simulink model "plant"  (R2022b)
settings: Solver=FixedStepAuto  StartTime=0.0  StopTime=10  FixedStep=0.00001  RelTol=1e-3
values from neighbouring files (symbols this model uses):
  ai = 0:0.03:20    [gain_schedule_co.m]
  Mi = 1.5:0.01:3    [gain_schedule_co.m]
undefined symbols (not defined in the file or in its folder): a_G0, a_G1, a_G2, a_G3, a_H0, a_H1, a_H2, a_H3, b_G0, b_G1, b_G2, b_G3, b_G4, b_H0, b_H1, b_H2, b_H3, b_H4, sigbuilder_block
libraries: cstblocks x2, SignalEditorBlockLib x1
settings Model: Creator=tomkeen  LastModifiedBy=tomkeen
settings SolverCC: AlgebraicLoopSolver=TrustRegion
settings DebuggingCC: UnconnectedInputMsg=warning  UnconnectedOutputMsg=warning  UnconnectedLineMsg=warning  SFMachineParentedDataDiag=warning
settings ModelReferenceCC: EnableRefExpFcnMdlSchedulingChecks=on
settings RTWCC: DLArmComputeVersion=19.05

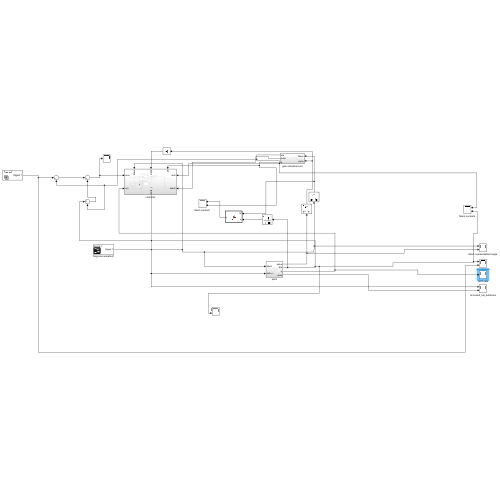
[thumbnail: Simulink's stored preview of the top-level diagram]
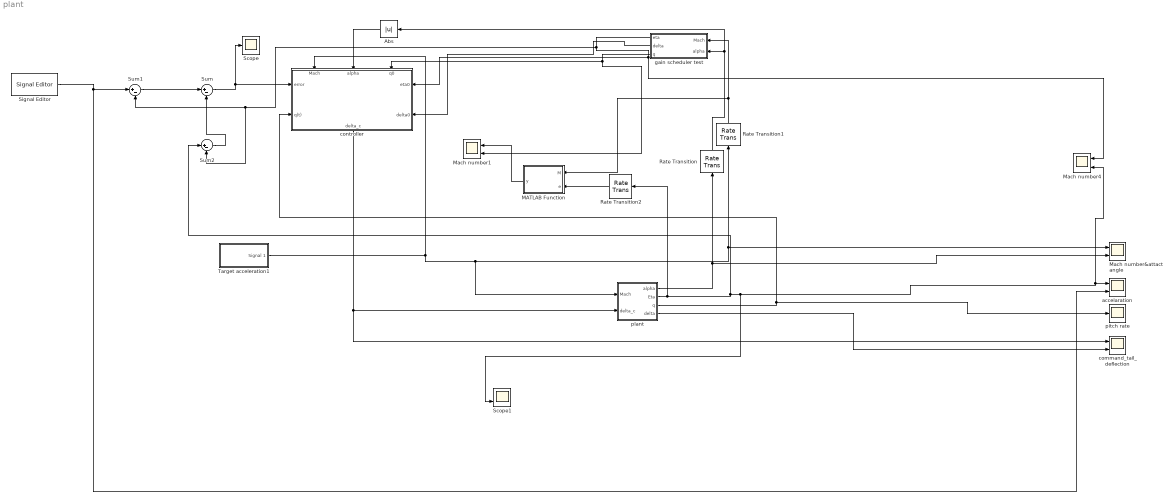
== system plant ==
  " pitch rate" : Scope
  Abs : Abs  SaturateOnIntegerOverflow=off
  MATLAB Function : MATLAB Function  TreatAsAtomicUnit=on
  Mach number&attact angle : Scope  NumInputPorts=2
  Mach number1 : Scope  NumInputPorts=2
  Mach number4 : Scope  NumInputPorts=2
  Rate Transition : RateTransition  OutPortSampleTime=0.001
  Rate Transition1 : RateTransition  OutPortSampleTime=0.001
  Rate Transition2 : RateTransition  OutPortSampleTime=0.0001
  Scope : Scope
  Scope1 : Scope  NumInputPorts=2
  Signal Editor : SignalEditorBlockLib/Signal Editor  FileName=signal.mat  ActiveScenario=Scenario  ActiveSignal=Signal 1  IsBus=off  OutputBusObjectStr=Bus: BusObject  SampleTime=0  Interpolate=off  ZeroCross=off  OutputAfterFinalValue=Setting to zero  Unit=inherit  PreserveSignalName=on
  Sum : Sum  Inputs=|+-
  Sum1 : Sum  Inputs=|+-
  Sum2 : Sum  Inputs=|+-
  Target acceleration1 : Subsystem  Tag=STV Subsys  LoadFcn=sigbuilder_block('load',[278.5 464.5 513.5 322.5 ]);  StartFcn=sigbuilder_block('start');  StopFcn=sigbuilder_block('stop');  ClipboardFcn=sigbuilder_block('clipboard');  mask(Sigbuilder block){tuvar=[0:10]}
      mask help: Simulink:masks:SigbuilderBlock_MD
      mask init:
      | if ~strcmp(get_param(bdroot(gcbh),'SimulationStatus'),'stopped') tuvar = sigbuilder_block('maskInit'); end
      settings: CopyFcn=sigbuilder_block('copy');  DeleteFcn=sigbuilder_block('delete');  ModelCloseFcn=sigbuilder_block('modelClose');  PreSaveFcn=sigbuilder_block('preSave');  PauseFcn=sigbuilder_block('pause');  ContinueFcn=sigbuilder_block('continue');  NameChangeFcn=sigbuilder_block('namechange');  OpenFcn=sigbuilder_block('open',[221 107.5 550.5 322.5 ]);  CloseFcn=sigbuilder_block('close');
      mask Display: plot(0, 0, 100, 100,[2, 2, 32, 32, 2], [68, 8, 8, 68, 68],[32, 2], [38, 38], [32, 19, 2],[53, 60, 44], [32, 17, 17, 2],[16, 16, 31, 31]);txt = getActiveGroup(gcbh);text(2, 100, txt,'verticalAlignment', 'top');
  accelaration : Scope  NumInputPorts=2
  command_tail_deflection : Scope  NumInputPorts=2
  controller : Subsystem
      settings: PortSchema="{\"entries\":[{\"content\":{\"sides\":[{\"content\":{\"connectorIds\":[\"In1\",\"In2\"]},\"type\":\"ConnectorPlacement.EquallySpacedRectSide\",\"uuid\":\"ccbd3968-3c34-4172-8982-2717baa6aaec\"},{\"content\":{\"connectorIds\":[\"In6\",\"In7\"],\"side\":\"RIGHT\"},\"type\":\"ConnectorPlacement.EquallySpacedRectSide\",\"uuid\":\"ff48a950-eb2b-4faf-a742-71355e33462e\"},{\"content\":{\"connectorIds\":[\"In3\",\"In4\",\"In5\"],\"side\":\"TOP\"},\"type\":\"ConnectorPlacement.EquallySpacedRectSide\",\"uuid\":\"543e7319-a8cd-4270-affa-865af0d15bcc\"},{\"content\":{\"connectorIds\":[\"Out1\"],\"side\":\"BOTTOM\"},\"type\":\"ConnectorPlacement.EquallySpacedRectSide\",\"uuid\":\"59242803-d082-430c-87a9-b5e2615a3fae\"}]},\"type\":\"ConnectorPlacement.EquallySpacedConnector\",\"uuid\":\"c7654354-e930-4276-ba78-f9f6fb08bf2c\"}],\"packageUris\":[\"http://schema.mathworks.com/mf0/Connector/R2020b\"],\"version\":\"1.0\"}"
  gain scheduler test : Subsystem
  plant : Subsystem
  wires:
  Target acceleration1/1(Signal 1) -> Rate Transition1/1, Mach number&attact angle/1, plant/1(Mach), controller/5(Mach)
  plant/2(Eta) -> Rate Transition2/1, Sum2/1, Scope1/2, Mach number4/2, accelaration/1
  plant/3(q) -> controller/7(q(t)), " pitch rate"/1
  plant/4(delta) -> command_tail_deflection/2
  gain scheduler test/2(delta) -> controller/2(delta0)
  gain scheduler test/3(q) -> controller/3(q0), Mach number1/2
  gain scheduler test/1(eta) -> controller/1(eta0), Mach number4/1, Sum2/2, Sum1/2
  Sum/1 -> Scope/1, controller/6(error)
  controller/1(delta_c) -> command_tail_deflection/1, plant/2(delta_c)
  Signal Editor/1 -> accelaration/2, Sum1/1
  Sum1/1 -> Sum/1
  Sum2/1 -> Sum/2
  Rate Transition/1 -> gain scheduler test/2(alpha), Abs/1
  Rate Transition1/1 -> gain scheduler test/1(Mach), MATLAB Function/1(M)
  plant/1(alpha) -> Rate Transition/1, Mach number&attact angle/2
  MATLAB Function/1(y) -> Mach number1/1
  Rate Transition2/1 -> MATLAB Function/2(e)
  Abs/1 -> controller/4(alpha)

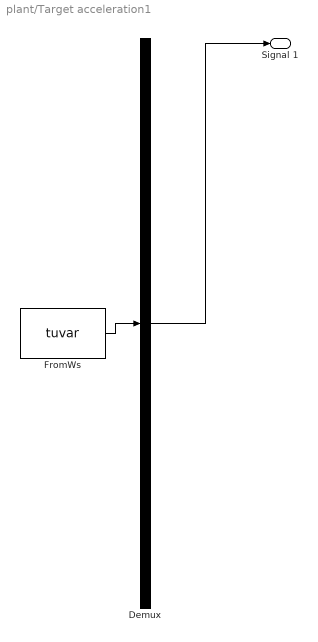
== system plant/Target acceleration1 ==
  Demux : Demux  Tag=STV Demux  Outputs=1
      settings: DisplayOption=none
  FromWs : FromWorkspace  Tag=STV FromWs  VariableName=tuvar
      SigBuilderData=|
      | common.afterFinalStr = 'Extrapolate'
      | common.sampleTime = 0
      | dataSet.timeRange = [0 10]
      | dataSet.name = 'Group 1'
      | sbobj.Groups.Name = 'Group 1'
      | sbobj.Groups.Signals.Name = 'Signal 1'
      | sbobj.Groups.Signals.XData = [0 10]
      | sbobj.Groups.Signals.YData = [2.69 2.48816513761]
  Signal 1 : Outport  Tag=STV Outport
  wires:
  Demux/1 -> Signal 1/1
  FromWs/1 -> Demux/1

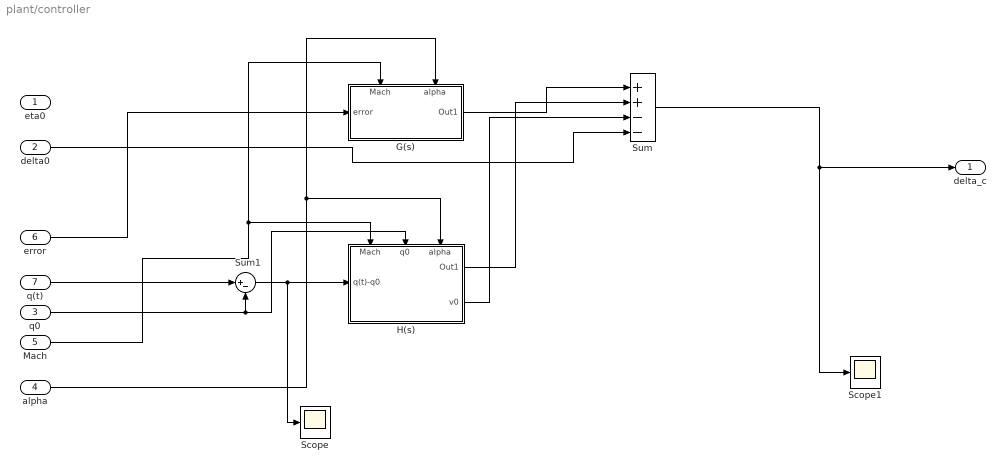
== system plant/controller ==
  eta0 : Inport
  delta0 : Inport  Port=2
  q0 : Inport  Port=3
  alpha : Inport  Port=4
  Mach : Inport  Port=5
  error : Inport  Port=6
  q(t) : Inport  Port=7
  G(s) : Subsystem
      settings: PortSchema="{\"entries\":[{\"content\":{\"sides\":[{\"content\":{\"connectorIds\":[\"In1\"]},\"type\":\"ConnectorPlacement.EquallySpacedRectSide\",\"uuid\":\"89c4dd89-01f0-41d8-90e7-82360ec46edc\"},{\"content\":{\"connectorIds\":[\"Out1\"],\"side\":\"RIGHT\"},\"type\":\"ConnectorPlacement.EquallySpacedRectSide\",\"uuid\":\"293521c5-f39c-474b-9224-6fe6832128f5\"},{\"content\":{\"connectorIds\":[\"In2\",\"In3\"],\"side\":\"TOP\"},\"type\":\"ConnectorPlacement.EquallySpacedRectSide\",\"uuid\":\"cd72ac66-ac52-4d27-85e4-85a309f5cd1a\"}]},\"type\":\"ConnectorPlacement.EquallySpacedConnector\",\"uuid\":\"92567c15-3faa-47ed-b120-3a292a4ff95e\"}],\"packageUris\":[\"http://schema.mathworks.com/mf0/Connector/R2020b\"],\"version\":\"1.0\"}"
  H(s) : Subsystem
      settings: PortSchema="{\"entries\":[{\"content\":{\"sides\":[{\"content\":{\"connectorIds\":[\"In1\"]},\"type\":\"ConnectorPlacement.EquallySpacedRectSide\",\"uuid\":\"89c4dd89-01f0-41d8-90e7-82360ec46edc\"},{\"content\":{\"connectorIds\":[\"Out1\",\"Out2\"],\"side\":\"RIGHT\"},\"type\":\"ConnectorPlacement.EquallySpacedRectSide\",\"uuid\":\"293521c5-f39c-474b-9224-6fe6832128f5\"},{\"content\":{\"connectorIds\":[\"In2\",\"In3\",\"In4\"],\"side\":\"TOP\"},\"type\":\"ConnectorPlacement.EquallySpacedRectSide\",\"uuid\":\"cd72ac66-ac52-4d27-85e4-85a309f5cd1a\"}]},\"type\":\"ConnectorPlacement.EquallySpacedConnector\",\"uuid\":\"92567c15-3faa-47ed-b120-3a292a4ff95e\"}],\"packageUris\":[\"http://schema.mathworks.com/mf0/Connector/R2020b\"],\"version\":\"1.0\"}"
  Scope : Scope
  Scope1 : Scope
  Sum : Sum  Inputs=|++--
  Sum1 : Sum  Inputs=|+-
  delta_c : Outport
  wires:
  G(s)/1(Out1) -> Sum/1
  H(s)/1(Out1) -> Sum/2
  Sum/1 -> Scope1/1, delta_c/1
  alpha/1 -> G(s)/3(alpha), H(s)/4(alpha)
  Mach/1 -> G(s)/2(Mach), H(s)/2(Mach)
  error/1 -> G(s)/1(error)
  q(t)/1 -> Sum1/1
  Sum1/1 -> Scope/1, H(s)/1(q(t)-q0)
  q0/1 -> H(s)/3(q0), Sum1/2
  H(s)/2(v0) -> Sum/3
  delta0/1 -> Sum/4

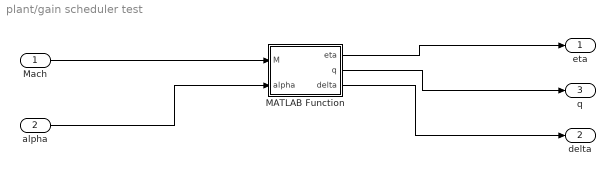
== system plant/gain scheduler test ==
  Mach : Inport
  alpha : Inport  Port=2
  MATLAB Function : MATLAB Function  TreatAsAtomicUnit=on
  eta : Outport
  delta : Outport  Port=2
  q : Outport  Port=3
  wires:
  Mach/1 -> MATLAB Function/1(M)
  alpha/1 -> MATLAB Function/2(alpha)
  MATLAB Function/1(eta) -> eta/1
  MATLAB Function/2(q) -> q/1
  MATLAB Function/3(delta) -> delta/1

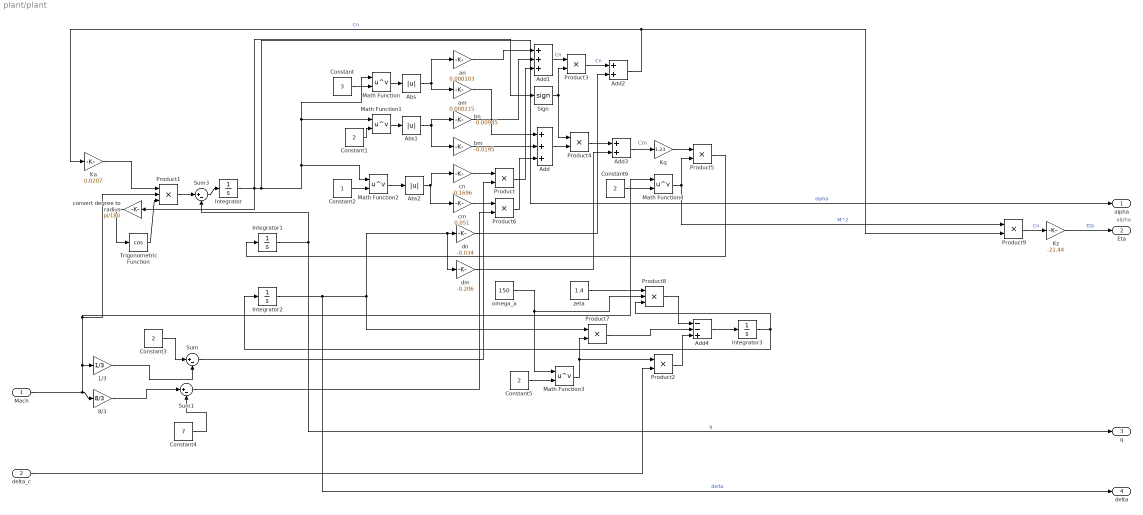
== system plant/plant ==
  note: alpha
  note: Cm
  Mach : Inport
  delta_c : Inport  Port=2
  1/3 : Gain  Gain=1/3
  8/3 : Gain  Gain=8/3
  Abs : Abs  SaturateOnIntegerOverflow=off
  Abs1 : Abs  SaturateOnIntegerOverflow=off
  Abs2 : Abs  SaturateOnIntegerOverflow=off
  Add : Sum  Inputs=+++
  Add1 : Sum  Inputs=+++
  Add2 : Sum
  Add3 : Sum
  Add4 : Sum  Inputs=--+
  Constant : Constant  Value=3
  Constant{1,3,5..6} (4 alike) : Constant  Value=2
  Constant2 : Constant
  Constant4 : Constant  Value=7
  Integrator{,1..3} (4 alike) : Integrator
  Ka : Gain  Gain=0.0207
  Kq : Gain  Gain=1.23
  Kz : Gain  Gain=-21.44
  Math Function{,1..4} (5 alike) : Math  Operator=pow
  Product{,2..7,9} (8 alike) : Product
  Product1 : Product  Inputs=3
  Product8 : Product  Inputs=3
  Sign : Signum
  Sum : Sum  Inputs=|+-
  Sum1 : Sum  Inputs=|+-
  Sum3 : Sum  Inputs=|+-
  Trigonometric Function : Trigonometry  Operator=cos
  am : Gain  Gain=0.000215
  an : Gain  Gain=0.000103
  bm : Gain  Gain=-0.0195
  bn : Gain  Gain=-0.00945
  cm : Gain  Gain=0.051
  cn : Gain  Gain=-0.1696
  convert degree to radius : Gain  Gain=pi/180
  dm : Gain  Gain=-0.206
  dn : Gain  Gain=-0.034
  omega_a : Constant  Value=150
  zeta : Constant  Value=1.4
  alpha : Outport
  Eta : Outport  Port=2
  q : Outport  Port=3
  delta : Outport  Port=4
  wires:
  Sign/1 -> Product4/1, Product3/2
  Product/1 -> Add1/3
  Integrator3/1 -> Integrator2/1, Product8/3
  Integrator1/1 -> q/1, Sum3/2  "q"
  Mach/1 -> Math Function4/1, Product1/2, 1/3/1, 8/3/1
  Sum/1 -> Product/2
  dm/1 -> Add3/2
  Add2/1 -> Product9/2, Ka/1  "Cn"
  Integrator2/1 -> delta/1, Product7/1, dm/1, dn/1  "delta"
  am/1 -> Add/1
  Abs/1 -> an/1, am/1
  Integrator/1 -> Sign/1, alpha/1, Math Function/1, Math Function1/1, Math Function2/1, convert degree to radius/1  "alpha"
  Abs1/1 -> bm/1, bn/1
  Ka/1 -> Product1/1
  Product4/1 -> Add3/1
  Add3/1 -> Kq/1
  Constant5/1 -> Math Function3/2
  Product5/1 -> Integrator1/1
  1/3/1 -> Sum/2
  Abs2/1 -> cm/1, cn/1
  cm/1 -> Product6/1
  Constant/1 -> Math Function/2
  zeta/1 -> Product8/1
  Constant3/1 -> Sum/1
  Product7/1 -> Add4/2
  Constant6/1 -> Math Function4/2
  an/1 -> Add1/1
  Product6/1 -> Add/3
  Constant4/1 -> Sum1/2
  bm/1 -> Add/2
  dn/1 -> Add2/2
  Math Function2/1 -> Abs2/1
  Add1/1 -> Product3/1  "Cn"
  Product1/1 -> Sum3/1
  Math Function1/1 -> Abs1/1
  Sum3/1 -> Integrator/1
  Math Function3/1 -> Product2/1, Product7/2
  omega_a/1 -> Product8/2, Math Function3/1
  Math Function/1 -> Abs/1
  Constant2/1 -> Math Function2/2
  cn/1 -> Product/1
  Add/1 -> Product4/2
  Trigonometric Function/1 -> Product1/3
  Product3/1 -> Add2/1  "Cn"
  bn/1 -> Add1/2
  delta_c/1 -> Product2/2
  8/3/1 -> Sum1/1
  Sum1/1 -> Product6/2
  Product8/1 -> Add4/1
  Product2/1 -> Add4/3
  Constant1/1 -> Math Function1/2
  Product9/1 -> Kz/1  "Cn"
  Math Function4/1 -> Product9/1, Product5/2  "M^2"
  Add4/1 -> Integrator3/1
  Kq/1 -> Product5/1
  Kz/1 -> Eta/1  "Eta"
  convert degree to radius/1 -> Trigonometric Function/1

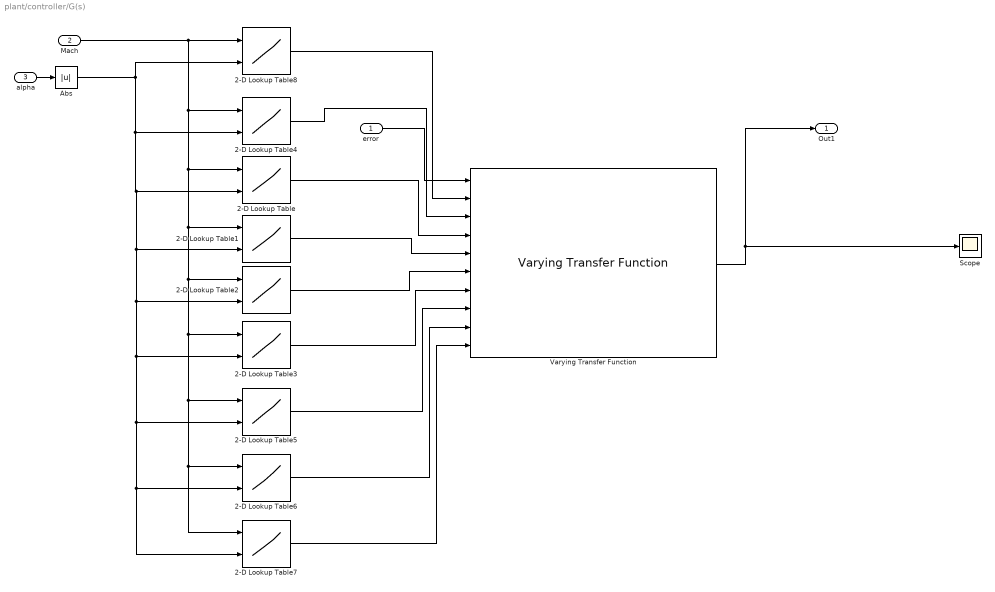
== system plant/controller/G(s) ==
  error : Inport
  Mach : Inport  Port=2
  alpha : Inport  Port=3
  2-D Lookup Table : Lookup_n-D  LookupTableObject=''  BreakpointsForDimension1=Mi  BreakpointsForDimension2=ai  BreakpointsForDimension1FirstPoint=10  BreakpointsForDimension2FirstPoint=10  BreakpointsForDimension1Spacing=12  BreakpointsForDimension2Spacing=12  IndexSearchMethod=Evenly spaced points  Table=b_G1  InterpMethod=Flat  DiagnosticForOutOfRangeInput=Error  InternalRulePriority=Speed  RndMeth=Simplest
      settings: InputPortMap=u0,u1
  2-D Lookup Table1 : Lookup_n-D  LookupTableObject=''  BreakpointsForDimension1=Mi  BreakpointsForDimension2=ai  BreakpointsForDimension1FirstPoint=10  BreakpointsForDimension2FirstPoint=10  BreakpointsForDimension1Spacing=12  BreakpointsForDimension2Spacing=12  IndexSearchMethod=Evenly spaced points  Table=a_G1  InterpMethod=Flat  DiagnosticForOutOfRangeInput=Error  InternalRulePriority=Speed  RndMeth=Simplest
      settings: InputPortMap=u0,u1
  2-D Lookup Table2 : Lookup_n-D  LookupTableObject=''  BreakpointsForDimension1=Mi  BreakpointsForDimension2=ai  BreakpointsForDimension1FirstPoint=10  BreakpointsForDimension2FirstPoint=10  BreakpointsForDimension1Spacing=12  BreakpointsForDimension2Spacing=12  IndexSearchMethod=Evenly spaced points  Table=b_G2  InterpMethod=Flat  DiagnosticForOutOfRangeInput=Error  InternalRulePriority=Speed  RndMeth=Simplest
      settings: InputPortMap=u0,u1
  2-D Lookup Table3 : Lookup_n-D  LookupTableObject=''  BreakpointsForDimension1=Mi  BreakpointsForDimension2=ai  BreakpointsForDimension1FirstPoint=10  BreakpointsForDimension2FirstPoint=10  BreakpointsForDimension1Spacing=12  BreakpointsForDimension2Spacing=12  IndexSearchMethod=Evenly spaced points  Table=a_G2  InterpMethod=Flat  DiagnosticForOutOfRangeInput=Error  InternalRulePriority=Speed  RndMeth=Simplest
      settings: InputPortMap=u0,u1
  2-D Lookup Table4 : Lookup_n-D  LookupTableObject=''  BreakpointsForDimension1=Mi  BreakpointsForDimension2=ai  BreakpointsForDimension1FirstPoint=10  BreakpointsForDimension2FirstPoint=10  BreakpointsForDimension1Spacing=12  BreakpointsForDimension2Spacing=12  IndexSearchMethod=Evenly spaced points  Table=a_G0  InterpMethod=Flat  DiagnosticForOutOfRangeInput=Error  InternalRulePriority=Speed  RndMeth=Simplest
      settings: InputPortMap=u0,u1
  2-D Lookup Table5 : Lookup_n-D  LookupTableObject=''  BreakpointsForDimension1=Mi  BreakpointsForDimension2=ai  BreakpointsForDimension1FirstPoint=10  BreakpointsForDimension2FirstPoint=10  BreakpointsForDimension1Spacing=12  BreakpointsForDimension2Spacing=12  IndexSearchMethod=Evenly spaced points  Table=b_G3  InterpMethod=Flat  DiagnosticForOutOfRangeInput=Error  InternalRulePriority=Speed  RndMeth=Simplest
      settings: InputPortMap=u0,u1
  2-D Lookup Table6 : Lookup_n-D  LookupTableObject=''  BreakpointsForDimension1=Mi  BreakpointsForDimension2=ai  BreakpointsForDimension1FirstPoint=10  BreakpointsForDimension2FirstPoint=10  BreakpointsForDimension1Spacing=12  BreakpointsForDimension2Spacing=12  IndexSearchMethod=Evenly spaced points  Table=a_G3  InterpMethod=Flat  DiagnosticForOutOfRangeInput=Error  InternalRulePriority=Speed  RndMeth=Simplest
      settings: InputPortMap=u0,u1
  2-D Lookup Table7 : Lookup_n-D  LookupTableObject=''  BreakpointsForDimension1=Mi  BreakpointsForDimension2=ai  BreakpointsForDimension1FirstPoint=10  BreakpointsForDimension2FirstPoint=10  BreakpointsForDimension1Spacing=12  BreakpointsForDimension2Spacing=12  IndexSearchMethod=Evenly spaced points  Table=b_G4  InterpMethod=Flat  DiagnosticForOutOfRangeInput=Error  InternalRulePriority=Speed  RndMeth=Simplest
      settings: InputPortMap=u0,u1
  2-D Lookup Table8 : Lookup_n-D  LookupTableObject=''  BreakpointsForDimension1=Mi  BreakpointsForDimension2=ai  BreakpointsForDimension1FirstPoint=10  BreakpointsForDimension2FirstPoint=10  BreakpointsForDimension1Spacing=12  BreakpointsForDimension2Spacing=12  IndexSearchMethod=Evenly spaced points  Table=b_G0  InterpMethod=Flat  DiagnosticForOutOfRangeInput=Error  InternalRulePriority=Speed  RndMeth=Simplest
      settings: InputPortMap=u0,u1
  Abs : Abs  SaturateOnIntegerOverflow=off
  Scope : Scope
  Varying Transfer Function : cstblocks/Linear Parameter Varying/Varying Transfer Function  N=4
  Out1 : Outport
  wires:
  error/1 -> Varying Transfer Function/1
  Varying Transfer Function/1 -> Out1/1, Scope/1
  2-D Lookup Table6/1 -> Varying Transfer Function/9
  2-D Lookup Table7/1 -> Varying Transfer Function/10
  2-D Lookup Table5/1 -> Varying Transfer Function/8
  2-D Lookup Table3/1 -> Varying Transfer Function/7
  2-D Lookup Table2/1 -> Varying Transfer Function/6
  2-D Lookup Table1/1 -> Varying Transfer Function/5
  2-D Lookup Table/1 -> Varying Transfer Function/4
  2-D Lookup Table4/1 -> Varying Transfer Function/3
  2-D Lookup Table8/1 -> Varying Transfer Function/2
  alpha/1 -> Abs/1
  Mach/1 -> 2-D Lookup Table8/1, 2-D Lookup Table4/1, 2-D Lookup Table1/1, 2-D Lookup Table2/1, 2-D Lookup Table3/1, 2-D Lookup Table5/1, 2-D Lookup Table6/1, 2-D Lookup Table7/1, 2-D Lookup Table/1
  Abs/1 -> 2-D Lookup Table8/2, 2-D Lookup Table4/2, 2-D Lookup Table1/2, 2-D Lookup Table2/2, 2-D Lookup Table3/2, 2-D Lookup Table5/2, 2-D Lookup Table6/2, 2-D Lookup Table7/2, 2-D Lookup Table/2

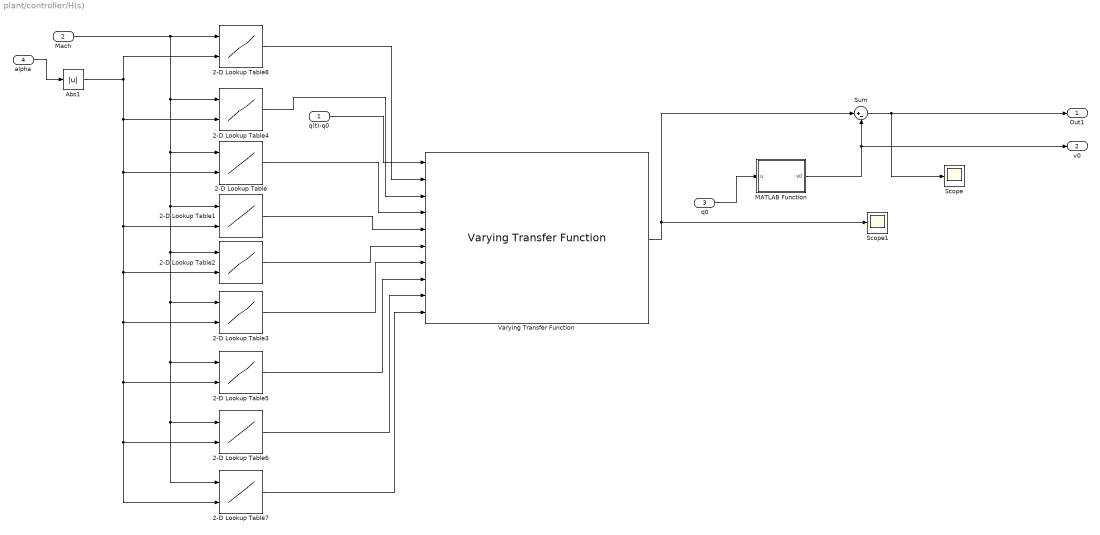
== system plant/controller/H(s) ==
  q(t)-q0 : Inport
  Mach : Inport  Port=2
  q0 : Inport  Port=3
  alpha : Inport  Port=4
  2-D Lookup Table : Lookup_n-D  LookupTableObject=''  BreakpointsForDimension1=Mi  BreakpointsForDimension2=ai  BreakpointsForDimension1FirstPoint=10  BreakpointsForDimension2FirstPoint=10  BreakpointsForDimension1Spacing=12  BreakpointsForDimension2Spacing=12  IndexSearchMethod=Evenly spaced points  Table=b_H1  InterpMethod=Flat  DiagnosticForOutOfRangeInput=Error  InternalRulePriority=Speed  RndMeth=Simplest
      settings: InputPortMap=u0,u1
  2-D Lookup Table1 : Lookup_n-D  LookupTableObject=''  BreakpointsForDimension1=Mi  BreakpointsForDimension2=ai  BreakpointsForDimension1FirstPoint=10  BreakpointsForDimension2FirstPoint=10  BreakpointsForDimension1Spacing=12  BreakpointsForDimension2Spacing=12  IndexSearchMethod=Evenly spaced points  Table=a_H1  InterpMethod=Flat  DiagnosticForOutOfRangeInput=Error  InternalRulePriority=Speed  RndMeth=Simplest
      settings: InputPortMap=u0,u1
  2-D Lookup Table2 : Lookup_n-D  LookupTableObject=''  BreakpointsForDimension1=Mi  BreakpointsForDimension2=ai  BreakpointsForDimension1FirstPoint=10  BreakpointsForDimension2FirstPoint=10  BreakpointsForDimension1Spacing=12  BreakpointsForDimension2Spacing=12  IndexSearchMethod=Evenly spaced points  Table=b_H2  InterpMethod=Flat  DiagnosticForOutOfRangeInput=Error  InternalRulePriority=Speed  RndMeth=Simplest
      settings: InputPortMap=u0,u1
  2-D Lookup Table3 : Lookup_n-D  LookupTableObject=''  BreakpointsForDimension1=Mi  BreakpointsForDimension2=ai  BreakpointsForDimension1FirstPoint=10  BreakpointsForDimension2FirstPoint=10  BreakpointsForDimension1Spacing=12  BreakpointsForDimension2Spacing=12  IndexSearchMethod=Evenly spaced points  Table=a_H2  InterpMethod=Flat  DiagnosticForOutOfRangeInput=Error  InternalRulePriority=Speed  RndMeth=Simplest
      settings: InputPortMap=u0,u1
  2-D Lookup Table4 : Lookup_n-D  LookupTableObject=''  BreakpointsForDimension1=Mi  BreakpointsForDimension2=ai  BreakpointsForDimension1FirstPoint=10  BreakpointsForDimension2FirstPoint=10  BreakpointsForDimension1Spacing=12  BreakpointsForDimension2Spacing=12  IndexSearchMethod=Evenly spaced points  Table=a_H0  InterpMethod=Flat  DiagnosticForOutOfRangeInput=Error  InternalRulePriority=Speed  RndMeth=Simplest
      settings: InputPortMap=u0,u1
  2-D Lookup Table5 : Lookup_n-D  LookupTableObject=''  BreakpointsForDimension1=Mi  BreakpointsForDimension2=ai  BreakpointsForDimension1FirstPoint=10  BreakpointsForDimension2FirstPoint=10  BreakpointsForDimension1Spacing=12  BreakpointsForDimension2Spacing=12  IndexSearchMethod=Evenly spaced points  Table=b_H3  InterpMethod=Flat  DiagnosticForOutOfRangeInput=Error  InternalRulePriority=Speed  RndMeth=Simplest
      settings: InputPortMap=u0,u1
  2-D Lookup Table6 : Lookup_n-D  LookupTableObject=''  BreakpointsForDimension1=Mi  BreakpointsForDimension2=ai  BreakpointsForDimension1FirstPoint=10  BreakpointsForDimension2FirstPoint=10  BreakpointsForDimension1Spacing=12  BreakpointsForDimension2Spacing=12  IndexSearchMethod=Evenly spaced points  Table=a_H3  InterpMethod=Flat  DiagnosticForOutOfRangeInput=Error  InternalRulePriority=Speed  RndMeth=Simplest
      settings: InputPortMap=u0,u1
  2-D Lookup Table7 : Lookup_n-D  LookupTableObject=''  BreakpointsForDimension1=Mi  BreakpointsForDimension2=ai  BreakpointsForDimension1FirstPoint=10  BreakpointsForDimension2FirstPoint=10  BreakpointsForDimension1Spacing=12  BreakpointsForDimension2Spacing=12  IndexSearchMethod=Evenly spaced points  Table=b_H4  InterpMethod=Flat  DiagnosticForOutOfRangeInput=Error  InternalRulePriority=Speed  RndMeth=Simplest
      settings: InputPortMap=u0,u1
  2-D Lookup Table8 : Lookup_n-D  LookupTableObject=''  BreakpointsForDimension1=Mi  BreakpointsForDimension2=ai  BreakpointsForDimension1FirstPoint=10  BreakpointsForDimension2FirstPoint=10  BreakpointsForDimension1Spacing=12  BreakpointsForDimension2Spacing=12  IndexSearchMethod=Evenly spaced points  Table=b_H0  InterpMethod=Flat  DiagnosticForOutOfRangeInput=Error  InternalRulePriority=Speed  RndMeth=Simplest
      settings: InputPortMap=u0,u1
  Abs1 : Abs  SaturateOnIntegerOverflow=off
  MATLAB Function : MATLAB Function  TreatAsAtomicUnit=on
  Scope : Scope
  Scope1 : Scope
  Sum : Sum  Inputs=|+-
  Varying Transfer Function : cstblocks/Linear Parameter Varying/Varying Transfer Function  N=4
  Out1 : Outport
  v0 : Outport  Port=2
  wires:
  q0/1 -> MATLAB Function/1(u)
  Sum/1 -> Scope/1, Out1/1
  MATLAB Function/1(v0) -> Sum/2, v0/1
  2-D Lookup Table4/1 -> Varying Transfer Function/3
  2-D Lookup Table/1 -> Varying Transfer Function/4
  2-D Lookup Table8/1 -> Varying Transfer Function/2
  2-D Lookup Table6/1 -> Varying Transfer Function/9
  alpha/1 -> Abs1/1
  2-D Lookup Table2/1 -> Varying Transfer Function/6
  2-D Lookup Table1/1 -> Varying Transfer Function/5
  2-D Lookup Table3/1 -> Varying Transfer Function/7
  Mach/1 -> 2-D Lookup Table8/1, 2-D Lookup Table4/1, 2-D Lookup Table1/1, 2-D Lookup Table2/1, 2-D Lookup Table3/1, 2-D Lookup Table5/1, 2-D Lookup Table6/1, 2-D Lookup Table7/1, 2-D Lookup Table/1
  q(t)-q0/1 -> Varying Transfer Function/1
  2-D Lookup Table7/1 -> Varying Transfer Function/10
  2-D Lookup Table5/1 -> Varying Transfer Function/8
  Varying Transfer Function/1 -> Sum/1, Scope1/1
  Abs1/1 -> 2-D Lookup Table8/2, 2-D Lookup Table4/2, 2-D Lookup Table1/2, 2-D Lookup Table2/2, 2-D Lookup Table3/2, 2-D Lookup Table5/2, 2-D Lookup Table6/2, 2-D Lookup Table7/2, 2-D Lookup Table/2

== matlab function plant/MATLAB Function ==
  data: M input; y output; e input
function y = fcn(M, e)

y = (3.0117e-5*e^3-0.58982*e)*(-0.1194*M^3+1.0984*M^2-3.6607*M+5.3222);

== matlab function plant/gain scheduler test/MATLAB Function ==
  data: eta output; q output; M input; alpha input; delta output
function [eta, q ,delta]= fcn(M, alpha)
%#codegen

Kz=21.44;
Ka=0.0207;
delta=-sign(alpha)*(0.000215*abs(alpha)^3-0.0195*abs(alpha)^2+0.051*abs(alpha)*(-7+8*M/3))/(-0.206)
alpha
Cn=sign(alpha)*(0.000103*abs(alpha)^3-0.00945*abs(alpha)^2-0.1696*abs(alpha)*(2-M/3))-0.034*delta;
q=-Ka*M*Cn*cos(alpha*pi/180);
eta=Kz*M^2*Cn

== matlab function plant/controller/H(s)/MATLAB Function ==
  data: u input; v0 output
function v0 = fcn(u)
zero_g2=[-158.09+158.05j;-158.09-158.05j; -104.21+107.35j;-104.21-107.35j; -0.60368];
pole_g2=[0; -56250; -1042.2; -144.97+163.15j;-144.97-163.15j; -104.16; -1.067];
gain_h2=[0.67619];
zero_h2=[0;-5000000; -1041.7; -104.12+107.34j; -104.12-107.34j; 14.625];
pole_h2=[0; -56250; -1042.2; -144.97+163.15j;-144.97-163.15j; -104.16; -1.067];

v0=2.*u
